simulink model "chuaTrackingUnexact_sim"  (R2024a)
settings: Solver=VariableStepAuto  StartTime=0.0  StopTime=t_sim  RelTol=1e-3
values from neighbouring files (symbols this model uses):
  gama = 2    [ChuaFL.m]    (also in chuaFLUnexact.m; chuaSMC.m)
  K = place(A, B, l_des)    [ChuaFL.m]    (also in chuaFLUnexact.m)
settings Model: Creator=lorenzo  LastModifiedBy=lorenzo

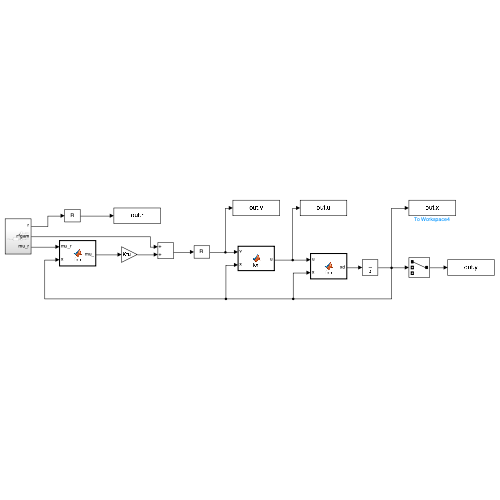
[thumbnail: Simulink's stored preview of the top-level diagram]
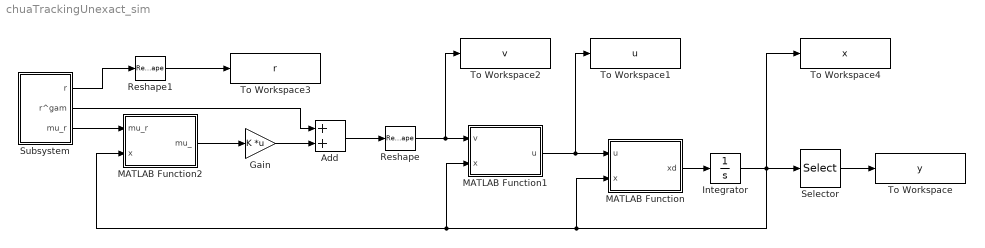
== system chuaTrackingUnexact_sim ==
  Add : Sum
  Gain : Gain  Gain=K  Multiplication=Matrix(K*u)
  Integrator : Integrator
  MATLAB Function : MATLAB Function  TreatAsAtomicUnit=on
  MATLAB Function1 : MATLAB Function  TreatAsAtomicUnit=on
  MATLAB Function2 : MATLAB Function  TreatAsAtomicUnit=on
  Reshape : Reshape  OutputDimensionality=Customize  OutputDimensions=[1]
  Reshape1 : Reshape  OutputDimensionality=Customize  OutputDimensions=[1]
  Selector : Selector  InputPortWidth=3  IndexOptions=Index vector (dialog)  Indices=1  OutputSizes=1
  Subsystem : Subsystem
  To Workspace : ToWorkspace  VariableName=y  SaveFormat=Timeseries  SampleTime=-1
  To Workspace1 : ToWorkspace  VariableName=u  SaveFormat=Timeseries  SampleTime=-1
  To Workspace2 : ToWorkspace  VariableName=v  SaveFormat=Timeseries  SampleTime=-1
  To Workspace3 : ToWorkspace  VariableName=r  SaveFormat=Timeseries  SampleTime=-1
  To Workspace4 : ToWorkspace  VariableName=x  SaveFormat=Timeseries  SampleTime=-1
  wires:
  MATLAB Function/1(xd) -> Integrator/1
  Integrator/1 -> To Workspace4/1, MATLAB Function1/2(x), MATLAB Function2/2(x), MATLAB Function/2(x), Selector/1
  MATLAB Function1/1(u) -> To Workspace1/1, MATLAB Function/1(u)
  MATLAB Function2/1(mu_) -> Gain/1
  Reshape/1 -> To Workspace2/1, MATLAB Function1/1(v)
  Add/1 -> Reshape/1
  Gain/1 -> Add/2
  Subsystem/3(mu_r) -> MATLAB Function2/1(mu_r)
  Subsystem/2(r^gam) -> Add/1
  Reshape1/1 -> To Workspace3/1
  Subsystem/1(r) -> Reshape1/1
  Selector/1 -> To Workspace/1

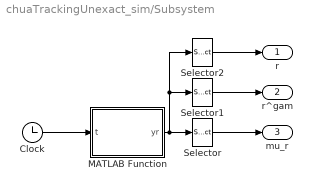
== system chuaTrackingUnexact_sim/Subsystem ==
  Clock : Clock
  MATLAB Function : MATLAB Function  TreatAsAtomicUnit=on
  Selector : Selector  InputPortWidth=gama+1  IndexOptions=Index vector (dialog)  Indices=1:gama  OutputSizes=1
  Selector1 : Selector  InputPortWidth=gama+1  IndexOptions=Index vector (dialog)  Indices=gama+1  OutputSizes=1
  Selector2 : Selector  InputPortWidth=gama+1  IndexOptions=Index vector (dialog)  Indices=1  OutputSizes=1
  r : Outport  VectorParamsAs1DForOutWhenUnconnected=off
  r^gam : Outport  Port=2  VectorParamsAs1DForOutWhenUnconnected=off
  mu_r : Outport  Port=3  VectorParamsAs1DForOutWhenUnconnected=off
  wires:
  Clock/1 -> MATLAB Function/1(t)
  Selector2/1 -> r/1
  MATLAB Function/1(yr) -> Selector2/1, Selector1/1, Selector/1
  Selector/1 -> mu_r/1
  Selector1/1 -> r^gam/1

== matlab function chuaTrackingUnexact_sim/MATLAB Function1 ==
  data: v input; u output; x input
function u = control_law(v,x)

alpha = 10.4;

rho_hat = -1.194*x(1) + 0.0422*x(1)^3;
rho_hatd = (633*x(1)^2)/5000 - 597/500; 

u = v/alpha - (x(1)-x(2)+x(3)-alpha*(x(2)-x(1)-rho_hat)*(1+rho_hatd));

== matlab function chuaTrackingUnexact_sim/MATLAB Function ==
  data: u input; xd output; x input
function xd = chua_plant(u,x)

R = 0.1; alpha = 10.4; beta = 16.5;
rho = -1.16*x(1) + 0.041*x(1)^3;

xd = [alpha*(x(2)-x(1)-rho);
 x(1)-x(2)+x(3)+u;
 -beta*x(2)-R*x(3)];

== matlab function chuaTrackingUnexact_sim/MATLAB Function2 ==
  data: mu_r input; x input; mu_ output
function mu_ = fcn(mu_r,x)

alpha = 10.4;
rho_hat = -1.194*x(1) + 0.0422*x(1)^3;
mu = [x(1); alpha*(x(2)-x(1)-rho_hat)];

mu_ = mu_r - mu;

== matlab function chuaTrackingUnexact_sim/Subsystem/MATLAB Function ==
  data: t input; yr output
function yr = ref_chua(t)

yr = [1.0;0.0;0.0];
end
